simulink model "F16AeroCoefficientsModel"  (R2024a)
settings: configuration reference "standardSILConfiguraitonParams" (kept outside this file)
undefined symbols (not defined in the file): alphaBkpts_nd, CZ, maxAilDefl_deg, maxRudderDefl_deg
libraries: AeroCoefficientLibrary x8, aerolibconvert2 x1
settings Model: Creator=jerem  LastModifiedBy=jerem
settings ConfigSetRef: SourceName=standardSILConfiguraitonParams  SourceLocation=Base Workspace

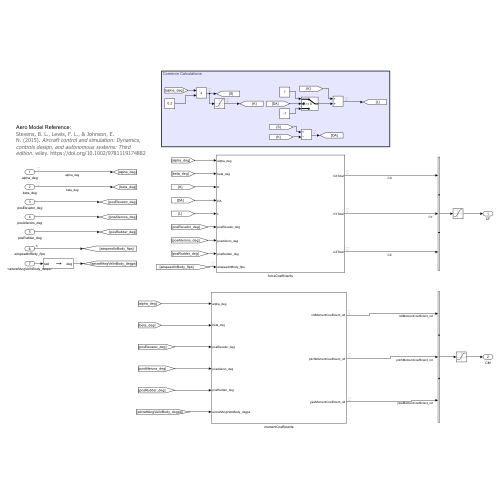
[thumbnail: Simulink's stored preview of the top-level diagram]
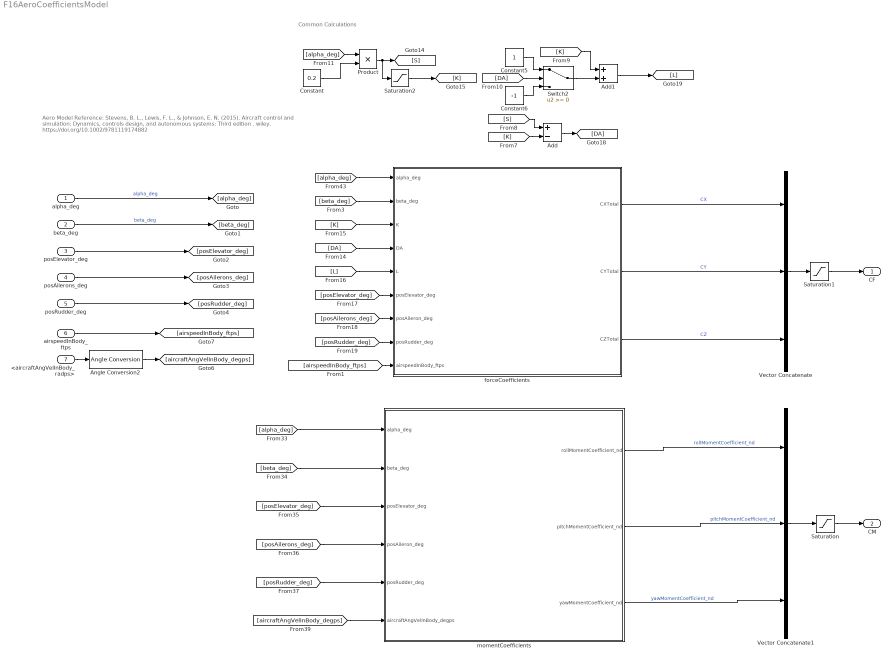
== system F16AeroCoefficientsModel ==
  note: Common Calculations
  note: Aero Model Reference:
      | Stevens, B. L., Lewis, F. L., & Johnson, E. N. (2015). Aircraft control and simulation: Dynamics, controls design, and autonomous systems: Third edition . wiley. https://doi.org/10.1002/9781119174882
  alpha_deg : Inport
  beta_deg : Inport  Port=2
  posElevator_deg : Inport  Port=3
  posAilerons_deg : Inport  Port=4
  posRudder_deg : Inport  Port=5
  airspeedInBody_ftps : Inport  Port=6  PortDimensions=[3]
  <aircraftAngVelInBody_radps> : Inport  Port=7
  Add : Sum  Inputs=+-
  Add1 : Sum
  Angle Conversion2 : aerolibconvert2/Angle Conversion  IU=rad  OU=deg
  Constant : Constant  Value=0.2
  Constant5 : Constant
  Constant6 : Constant  Value=-1
  Product : Product
  Saturation : Saturate  UpperLimit=3  LowerLimit=-3
  Saturation1 : Saturate  UpperLimit=30  LowerLimit=-30
  Saturation2 : Saturate  UpperLimit=8  LowerLimit=-1
  Switch2 : Switch  SaturateOnIntegerOverflow=off  InputSameDT=off
  Vector Concatenate : Concatenate  NumInputs=3
  Vector Concatenate1 : Concatenate  NumInputs=3
  forceCoefficients : Subsystem
  momentCoefficients : Subsystem
  CF : Outport
  CM : Outport  Port=2
  wires:
  alpha_deg/1 -> [alpha_deg]  "alpha_deg"
  Vector Concatenate/1 -> Saturation1/1
  [posAilerons_deg] -> momentCoefficients/4(posAileron_deg)
  [beta_deg] -> momentCoefficients/2(beta_deg)
  [K] -> Add/2
  [aircraftAngVelInBody_degps] -> momentCoefficients/6(aircraftAngVelInBody_degps)
  momentCoefficients/1(rollMomentCoefficient_nd) -> Vector Concatenate1/1  "rollMomentCoefficient_nd"
  [posRudder_deg] -> momentCoefficients/5(posRudder_deg)
  [S] -> Add/1
  [alpha_deg] -> Product/1
  [posAilerons_deg] -> forceCoefficients/7(posAileron_deg)
  [K] -> forceCoefficients/3(K)
  [posRudder_deg] -> forceCoefficients/8(posRudder_deg)
  [posElevator_deg] -> forceCoefficients/6(posElevator_deg)
  [K] -> Add1/1
  Add1/1 -> [L]
  Product/1 -> Saturation2/1, [S]
  Constant6/1 -> Switch2/3
  Constant5/1 -> Switch2/1
  [beta_deg] -> forceCoefficients/2(beta_deg)
  airspeedInBody_ftps/1 -> [airspeedInBody_ftps]
  forceCoefficients/1(CXTotal) -> Vector Concatenate/1  "CX"
  <aircraftAngVelInBody_radps>/1 -> Angle Conversion2/1
  posAilerons_deg/1 -> [posAilerons_deg]
  [DA] -> forceCoefficients/4(DA)
  forceCoefficients/3(CZTotal) -> Vector Concatenate/3  "CZ"
  [DA] -> Switch2/2
  Add/1 -> [DA]
  Vector Concatenate1/1 -> Saturation/1
  Constant/1 -> Product/2
  momentCoefficients/2(pitchMomentCoefficient_nd) -> Vector Concatenate1/2  "pitchMomentCoefficient_nd"
  [alpha_deg] -> momentCoefficients/1(alpha_deg)
  posElevator_deg/1 -> [posElevator_deg]
  posRudder_deg/1 -> [posRudder_deg]
  momentCoefficients/3(yawMomentCoefficient_nd) -> Vector Concatenate1/3  "yawMomentCoefficient_nd"
  [L] -> forceCoefficients/5(L)
  [posElevator_deg] -> momentCoefficients/3(posElevator_deg)
  beta_deg/1 -> [beta_deg]  "beta_deg"
  forceCoefficients/2(CYTotal) -> Vector Concatenate/2  "CY"
  Switch2/1 -> Add1/2
  [alpha_deg] -> forceCoefficients/1(alpha_deg)
  Saturation/1 -> CM/1
  Saturation1/1 -> CF/1
  Saturation2/1 -> [K]
  Angle Conversion2/1 -> [aircraftAngVelInBody_degps]
  [airspeedInBody_ftps] -> forceCoefficients/9(airspeedInBody_ftps)

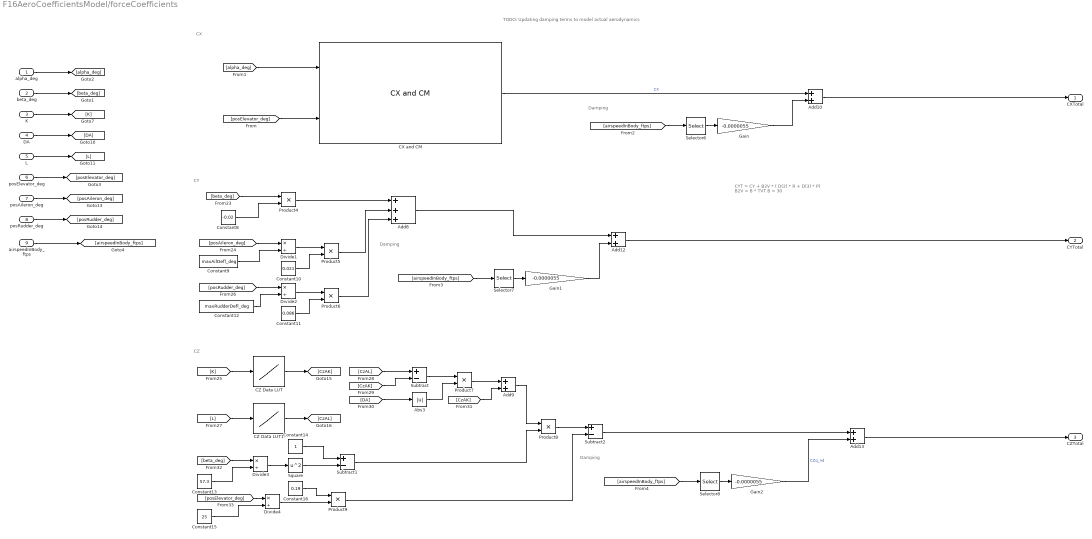
== system F16AeroCoefficientsModel/forceCoefficients ==
  note: TODO: Updating damping terms to model actual aerodynamics
  note: CZ
  note: CY
  note: CX
  note: CYT = CY + B2V * ( D(2) * R + D(3) * P)
      |
      | B2V = B * TVT
      | B = 30
  note: Damping
  note: Damping
  note: Damping
  alpha_deg : Inport
  beta_deg : Inport  Port=2
  K : Inport  Port=3
  DA : Inport  Port=4
  L : Inport  Port=5
  posElevator_deg : Inport  Port=6
  posAileron_deg : Inport  Port=7
  posRudder_deg : Inport  Port=8
  airspeedInBody_ftps : Inport  Port=9
  Abs3 : Abs  SaturateOnIntegerOverflow=off
  Add{9..10,12..13} (4 alike) : Sum
  Add8 : Sum  Inputs=+++
  CX and CM : AeroCoefficientLibrary/CX and CM  aeroData=CX  alphaBkpts_nd=alphaBkpts_nd  elevBkpts_nd=elevBkpts_nd
  CZ Data LUT : Lookup_n-D  NumberOfTableDimensions=1  BreakpointsForDimension1=alphaBkpts_nd  Table=CZ  ExtrapMethod=Clip  DiagnosticForOutOfRangeInput=Warning  InternalRulePriority=Speed  RndMeth=Simplest
  CZ Data LUT1 : Lookup_n-D  NumberOfTableDimensions=1  BreakpointsForDimension1=alphaBkpts_nd  Table=CZ  ExtrapMethod=Clip  DiagnosticForOutOfRangeInput=Warning  InternalRulePriority=Speed  RndMeth=Simplest
  Constant10 : Constant  Value=0.021
  Constant11 : Constant  Value=0.086
  Constant12 : Constant  Value=maxRudderDefl_deg
  Constant13 : Constant  Value=57.3
  Constant14 : Constant
  Constant15 : Constant  Value=25
  Constant16 : Constant  Value=0.19
  Constant8 : Constant  Value=-0.02
  Constant9 : Constant  Value=maxAilDefl_deg
  Divide{1..4} (4 alike) : Product  Inputs=*/
  Gain : Gain  Gain=-0.0000055
  Gain1 : Gain  Gain=-0.0000055
  Gain2 : Gain  Gain=-0.0000055
  Product{4..9} (6 alike) : Product
  Selector6 : Selector  InputPortWidth=3  IndexOptions=Index vector (dialog)  Indices=1  OutputSizes=1
  Selector7 : Selector  InputPortWidth=3  IndexOptions=Index vector (dialog)  Indices=2  OutputSizes=1
  Selector8 : Selector  InputPortWidth=3  IndexOptions=Index vector (dialog)  Indices=3  OutputSizes=1
  Square : Math  Operator=square
  Subtract : Sum  Inputs=+-
  Subtract1 : Sum  Inputs=+-
  Subtract2 : Sum  Inputs=+-
  CXTotal : Outport
  CYTotal : Outport  Port=2
  CZTotal : Outport  Port=3
  wires:
  beta_deg/1 -> [beta_deg]
  posElevator_deg/1 -> [posElevator_deg]
  K/1 -> [K]
  DA/1 -> [DA]
  L/1 -> [L]
  [beta_deg] -> Product4/1
  Constant8/1 -> Product4/2
  Product4/1 -> Add8/1
  posAileron_deg/1 -> [posAileron_deg]
  [posAileron_deg] -> Divide1/1
  Constant9/1 -> Divide1/2
  Divide1/1 -> Product5/1
  Constant10/1 -> Product5/2
  Product5/1 -> Add8/2
  Constant12/1 -> Divide2/2
  [posRudder_deg] -> Divide2/1
  Divide2/1 -> Product6/1
  Constant11/1 -> Product6/2
  posRudder_deg/1 -> [posRudder_deg]
  Product6/1 -> Add8/3
  [K] -> CZ Data LUT/1
  CZ Data LUT/1 -> [CzAK]
  CZ Data LUT1/1 -> [CzAL]
  [L] -> CZ Data LUT1/1
  [CzAK] -> Subtract/2
  [CzAL] -> Subtract/1
  Subtract/1 -> Product7/1
  [DA] -> Abs3/1
  Abs3/1 -> Product7/2
  Product7/1 -> Add9/1
  [CzAK] -> Add9/2
  [beta_deg] -> Divide3/1
  Constant13/1 -> Divide3/2
  Divide3/1 -> Square/1
  Square/1 -> Subtract1/2
  Constant14/1 -> Subtract1/1
  Subtract1/1 -> Product8/2
  Add9/1 -> Product8/1
  Product8/1 -> Subtract2/1
  Constant15/1 -> Divide4/2
  [posElevator_deg] -> Divide4/1
  Divide4/1 -> Product9/2
  Constant16/1 -> Product9/1
  Product9/1 -> Subtract2/2
  CX and CM/1 -> Add10/1  "CX"
  Selector6/1 -> Gain/1
  Add10/1 -> CXTotal/1
  Add8/1 -> Add12/1
  Add12/1 -> CYTotal/1
  Subtract2/1 -> Add13/1
  Gain2/1 -> Add13/2  "CZq_nd"
  [posElevator_deg] -> CX and CM/2
  alpha_deg/1 -> [alpha_deg]
  [alpha_deg] -> CX and CM/1
  Add13/1 -> CZTotal/1
  Gain1/1 -> Add12/2
  airspeedInBody_ftps/1 -> [airspeedInBody_ftps]
  [airspeedInBody_ftps] -> Selector6/1
  Gain/1 -> Add10/2
  Selector7/1 -> Gain1/1
  [airspeedInBody_ftps] -> Selector7/1
  Selector8/1 -> Gain2/1
  [airspeedInBody_ftps] -> Selector8/1

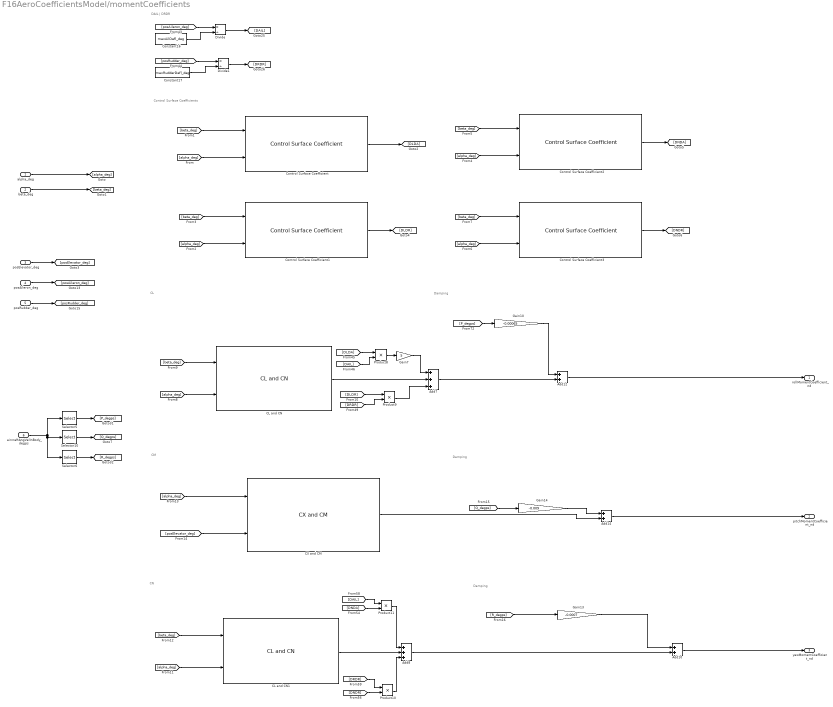
== system F16AeroCoefficientsModel/momentCoefficients ==
  note: Damping
  note: CL
  note: Control Surface Coefficients
  note: CN
  note: CM
  note: DAIL | DRDR
  note: Damping
  note: Damping
  alpha_deg : Inport
  beta_deg : Inport  Port=2
  posElevator_deg : Inport  Port=3
  posAileron_deg : Inport  Port=4
  posRudder_deg : Inport  Port=5
  aircraftAngVelInBody_degps : Inport  Port=6
  Add10 : Sum
  Add12 : Sum
  Add14 : Sum
  Add7 : Sum  Inputs=+++
  Add8 : Sum  Inputs=+++
  CL and CN : AeroCoefficientLibrary/CL and CN  aeroData=CL  betaBkpts_nd=betaBkpts_nd  alphaBkpts_nd=alphaBkpts_nd
      link override From10: GotoTag=Kfinal
      link override From26: GotoTag=Kfinal
  CL and CN1 : AeroCoefficientLibrary/CL and CN  aeroData=CN  betaBkpts_nd=betaBkpts_nd  alphaBkpts_nd=alphaBkpts_nd
  CX and CM : AeroCoefficientLibrary/CX and CM  aeroData=CM  alphaBkpts_nd=alphaBkpts_nd  elevBkpts_nd=elevBkpts_nd
  Constant16 : Constant  Value=maxAilDefl_deg
  Constant17 : Constant  Value=maxRudderDefl_deg
  Control Surface Coefficient : AeroCoefficientLibrary/Control Surface Coefficient  aeroData=dLdAil  betaBkpts_nd=betaBkpts_nd  alphaBkpts_nd=alphaBkpts_nd
  Control Surface Coefficient1 : AeroCoefficientLibrary/Control Surface Coefficient  aeroData=dLdRud  betaBkpts_nd=betaBkpts_nd  alphaBkpts_nd=alphaBkpts_nd
  Control Surface Coefficient2 : AeroCoefficientLibrary/Control Surface Coefficient  aeroData=dNdAil  betaBkpts_nd=betaBkpts_nd  alphaBkpts_nd=alphaBkpts_nd
  Control Surface Coefficient3 : AeroCoefficientLibrary/Control Surface Coefficient  aeroData=dNdRud  betaBkpts_nd=betaBkpts_nd  alphaBkpts_nd=alphaBkpts_nd
  Divide : Product  Inputs=*/
  Divide1 : Product  Inputs=*/
  Gain10 : Gain  Gain=-0.00065
  Gain13 : Gain  Gain=-0.0007
  Gain14 : Gain  Gain=-0.009
  Gain7 : Gain  Gain=5
  Product{8..11} (4 alike) : Product
  Selector10 : Selector  InputPortWidth=3  IndexOptions=Index vector (dialog)  Indices=2  OutputSizes=1
  Selector5 : Selector  InputPortWidth=3  IndexOptions=Index vector (dialog)  Indices=1  OutputSizes=1
  Selector6 : Selector  InputPortWidth=3  IndexOptions=Index vector (dialog)  Indices=3  OutputSizes=1
  rollMomentCoefficient_nd : Outport
  pitchMomentCoefficient_nd : Outport  Port=2
  yawMomentCoefficient_nd : Outport  Port=3
  wires:
  alpha_deg/1 -> [alpha_deg]
  beta_deg/1 -> [beta_deg]
  posElevator_deg/1 -> [posElevator_deg]
  posAileron_deg/1 -> [posAileron_deg]
  posRudder_deg/1 -> [posRudder_deg]
  [posAileron_deg] -> Divide/1
  Constant16/1 -> Divide/2
  Divide/1 -> [DAIL]
  [posRudder_deg] -> Divide1/1
  Constant17/1 -> Divide1/2
  Divide1/1 -> [DRDR]
  [DNDR] -> Product10/2
  [DRDR] -> Product10/1
  [DNDA] -> Product11/2
  [DAIL] -> Product11/1
  Product10/1 -> Add8/3
  Selector5/1 -> [P_degps]
  Selector6/1 -> [R_degps]
  aircraftAngVelInBody_degps/1 -> Selector10/1, Selector6/1, Selector5/1
  Add10/1 -> yawMomentCoefficient_nd/1
  [alpha_deg] -> Control Surface Coefficient/2
  [beta_deg] -> Control Surface Coefficient/1
  [beta_deg] -> Control Surface Coefficient1/1
  [alpha_deg] -> Control Surface Coefficient1/2
  [beta_deg] -> Control Surface Coefficient2/1
  [alpha_deg] -> Control Surface Coefficient2/2
  [beta_deg] -> Control Surface Coefficient3/1
  [alpha_deg] -> Control Surface Coefficient3/2
  Control Surface Coefficient1/1 -> [DLDR]
  Control Surface Coefficient2/1 -> [DNDA]
  Control Surface Coefficient3/1 -> [DNDR]
  [beta_deg] -> CL and CN/1
  [alpha_deg] -> CL and CN/2
  [DLDA] -> Product8/1
  [P_degps] -> Gain10/1
  Add7/1 -> Add12/2
  [DRDR] -> Product9/2
  Product9/1 -> Add7/3
  Product8/1 -> Gain7/1
  [DLDR] -> Product9/1
  [DAIL] -> Product8/2
  Add12/1 -> rollMomentCoefficient_nd/1
  CL and CN/1 -> Add7/2
  [beta_deg] -> CL and CN1/1
  [alpha_deg] -> CL and CN1/2
  Product11/1 -> Add8/1
  CL and CN1/1 -> Add8/2
  [alpha_deg] -> CX and CM/1
  [posElevator_deg] -> CX and CM/2
  Control Surface Coefficient/1 -> [DLDA]
  Gain7/1 -> Add7/1
  Add14/1 -> pitchMomentCoefficient_nd/1
  Add8/1 -> Add10/2
  Gain10/1 -> Add12/1
  Gain13/1 -> Add10/1
  Selector10/1 -> [Q_degps]
  [Q_degps] -> Gain14/1
  Gain14/1 -> Add14/1
  [R_degps] -> Gain13/1
  CX and CM/1 -> Add14/2
